simulink model "BMS_V4"  (R2017b)
settings: Solver=FixedStepDiscrete  StartTime=0.0  StopTime=inf  FixedStep=BASETIME  RelTol=1e-3  EnableMultiTasking=on
values from neighbouring files (symbols this model uses):
  AKT_BALANCE = uint16(8)    [BMS_V4_config.m]
  BALANCE = uint16(4)    [BMS_V4_config.m]
  BALANCE_RESISTOR = int32(5)    [BMS_V4_config.m]
  BALANCE_VEC = uint16(8)    [BMS_V4_config.m]
  CELL_SOC = uint16(7)    [BMS_V4_config.m]
  CELL_STATE = uint16(3)    [BMS_V4_config.m]
  CELL_TEMPERATURE = uint16(6)    [BMS_V4_config.m]
  CELL_VOLTAGE = uint16(5)    [BMS_V4_config.m]
  CELLACTBITFIELD = hex2dec('300')    [BMS_V4_config.m]
  CELLDEACTBITFIELD = hex2dec('100')    [BMS_V4_config.m]
  CELLT_BURST = uint16(6)    [BMS_V4_config.m]
  CELLV_BURST = uint16(5)    [BMS_V4_config.m]
  CLK_CYC_timer_1 = 586    [BMS_V4_config.m]
  CLK_CYC_timer_2 = 5860    [BMS_V4_config.m]
  CLK_CYC_timer_3 = 280    [BMS_V4_config.m]
  CLK_CYC_timer_4 = 586*100    (= 58600)    [BMS_V4_config.m]
  CLK_CYC_timer_5 = 5800*2    (= 11600)    [BMS_V4_config.m]
  CLK_CYC_timer_6 = 320    [BMS_V4_config.m]
  CN_CELLS = int32(40*3600)    [BMS_V4_config.m]
  CONTACTOR = uint16(1)    [BMS_V4_config.m]
  CONTACTOR_LOCKED = uint16(0)    [BMS_V4_config.m]
  CONTACTOR_UNLOCKED = uint16(1)    [BMS_V4_config.m]
  DEBUG_SEND_STATES = uint16(hex2dec('01'))    [BMS_V4_config.m]
  DELTA_SOC_BALANCE = int32(5*1e6)    [BMS_V4_config.m]
  DELTA_SOC_BALANCE_OFF = int32(1*1e5)    [BMS_V4_config.m]
  DETERMINE_MODEL_PARAMETER_ACT = uint16(100)    [BMS_V4_config.m]
  DETERMINE_MODEL_PARAMETER_SCC = uint16(101)    [BMS_V4_config.m]
  ERROR = uint16(1)    [BMS_V4_config.m]
  EXTERN_SIGNALS = uint16(1)    [BMS_V4_config.m]
  FREQUENCY_STEPS = uint16([25 50 75 100 150 250 500 750                                      1000 1500 2500 5000 7500                                      10010 10015 10025 10050 10075                                      10100 10150 10250 10500 10750                                      11000 11500])    [BMS_V4_config.m]
  GET_IMAG_PART_MFC = uint16(9)    [BMS_V4_config.m]
  GET_IMAG_PART_MSF = uint16(4)    [BMS_V4_config.m]
  GET_REAL_PART_MFC = uint16(8)    [BMS_V4_config.m]
  GET_REAL_PART_MSF = uint16(3)    [BMS_V4_config.m]
  IMU = uint16(7)    [BMS_V4_config.m]
  IMU_AMP_OFF = uint16(5)    [BMS_V4_config.m]
  IMU_DATA_READ_LOCUS_ACT = uint16(6)    [BMS_V4_config.m]
  IMU_DATA_READ_LOCUS_SCC = uint16(7)    [BMS_V4_config.m]
  IMU_DEBUG = uint16(9)    [BMS_V4_config.m]
  IMU_GET_DATA_MFC = uint16(8)    [BMS_V4_config.m]
  IMU_GET_DATA_MSF = uint16(3)    [BMS_V4_config.m]
  IMU_OFFSET_POLLING = uint16(11)    [BMS_V4_config.m]
  IMU_POLLING = uint16(2)    [BMS_V4_config.m]
  IMU_POWER = uint16(10)    [BMS_V4_config.m]
  IMU_SEND_IMAG = uint16(11)    [BMS_V4_config.m]
  IMU_SEND_REAL = uint16(10)    [BMS_V4_config.m]
  INDEX_IMAGPART = uint16(2)    [BMS_V4_config.m]
  INDEX_REALPART = uint16(1)    [BMS_V4_config.m]
  INFO = uint16(2)    [BMS_V4_config.m]
  INIT_OFFSET_AMPLITUDE = uint16(2)    [BMS_V4_config.m]
  LINE_CURRENT = uint16(3)    [BMS_V4_config.m]
  LINE_CURRENT_CANA = uint16(4)    [BMS_V4_config.m]
  LINE_CURRENT_SWITCH_THRESHOLD = int32(2*1e6)    [BMS_V4_config.m]
  NUM_OF_CELLS = uint16(16)    [BMS_V4_config.m]
  NUM_OF_FREQUENCIES_PSO = uint16(14)    [BMS_V4_config.m]
  NUM_OF_LINES = uint16(1)    [BMS_V4_config.m]
  NUM_OF_PARAMETER = single(5)    [BMS_V4_config.m]
  NUM_OF_SOC_POINTS = uint16(110)    [BMS_V4_config.m]
  P_L_BOUND = single([0.05;0.01;0.1;0.01;0.1])    [BMS_V4_config.m]
  P_U_BOUND = single([0.50;0.20;0.9;0.06;60])    [BMS_V4_config.m]
  PARA_ACT_SEND = uint16(101)    [BMS_V4_config.m]
  PARA_DATA_STORE_ACT = uint16(8)    [BMS_V4_config.m]
  PARA_DATA_STORE_SCC = uint16(9)    [BMS_V4_config.m]
  PARA_SCC_SEND = uint16(102)    [BMS_V4_config.m]
  PARTICLE_INIT = single(create_startparticle(P_L_BOUND,P_U_BOUND,NUM_OF_PARTICLE))    [BMS_V4_config.m]
  POLACT = hex2dec('00000BFF')    [BMS_V4_config.m]
  POLDEACT = hex2dec('000008FF')    [BMS_V4_config.m]
  PSO_PARA_DEBUG = uint16(13)    [BMS_V4_config.m]
  REQUEST_SOC_REF = uint16(1000)    [BMS_V4_config.m]
  SCALE_FACTOR_CH1 = single(0.66666666)    [BMS_V4_config.m]
  SCALE_FACTOR_CH2 = single(0.66666666)    [BMS_V4_config.m]
  SEND_CELL_SOC_ABS = uint16(199)    [BMS_V4_config.m]
  SHUT_DOWN_BALANCE_OFF = uint16(3)    [BMS_V4_config.m]
  SHUT_DOWN_BALANCE_ON = uint16(2)    [BMS_V4_config.m]
  START_IMU_MSL = uint16(3)    [BMS_V4_config.m]
  START_IMU_SCC = uint16(1)    [BMS_V4_config.m]
  SWITCH_IMU_OFF = uint16(2)    [BMS_V4_config.m]
  SWITCH_IMU_ON = uint16(1)    [BMS_V4_config.m]
  SWITCH_IMU_ON_OFF = uint16(4)    [BMS_V4_config.m]
  SYSTEM_DEBUG = uint16(12)    [BMS_V4_config.m]
  TIMEOUT_CANA = uint32(5000)    [BMS_V4_config.m]
  TIMEOUT_GATEWAY = uint32(500)    [BMS_V4_config.m]
  TS_SOC = single(0.010)    [BMS_V4_config.m]
  WARNING = uint16(2)    [BMS_V4_config.m]
libraries: c280xlib x44, c2833xlib x5, simulink x2, c2000lib x1, idelinklib_common x1
(part 6 of 8)

== stateflow chart BMS_V4/IMU_control ==
  state IMU
    state IMU_control [parallel]
      settings: executionOrder=1
      state init_
        en:
        imu_state=uint16(IMU_INIT);
        //imu_function = uint16(0);
      state IMU_start_slave
        state power_on_imu
          en:
          imu_state = IMU_POWER_ON;
          //balance disable
          imu_request = IMU_POWER;
          imu_in_progress=true;
          [imu_CAN_low, imu_CAN_high] = IMU_on_off(SWITCH_IMU_ON);
          gateway_request[IMU - uint16(1)] = true;
        state wait
          en:
        state init_offset_amplitude
          en:
          imu_on_off = true;
          imu_state = IMU_INIT_AMP_OFF;
          imu_request = IMU_AMP_OFF;
          [imu_CAN_low, imu_CAN_high] = IMU_set_offset_amplitude(imu_offset,imu_amplitude);
          //[imu_CAN_low, imu_CAN_high] = IMU_set_offset_amplitude(uint16(2000),uint16(500));
          gateway_request[IMU - uint16(1)] = true;
        power_on_imu -> wait : [imu_request_succed == true]
            | //clear MSG flag
            | {imu_request_succed = false;
            | imu_on_off = true;}
        wait -> init_offset_amplitude : after(TIMER_IMU_START_UP,sec)
      state reset
        imu_function = uint16(0);
      state IMU_msl
        // meas single locus
        state set_offset_on
          en:
          imu_state=MSL_SWITCH_OFFSET_ON;
          offset_flag = SWITCH_OFFSET_ON;
          send(IMU_OFFSET,IMU.IMU_offset_on_off);
        state time_for_transient_response
          en:
        state start_locus_measurement
          en:
          IMU_save_act_imu_soc();
          imu_state = MSL_START_LOCUS_MEAS;
          send(IMU_MEAS_LOCUS,IMU.IMU_meas_locus);
        state set_offset_off
          en:
          imu_state=MSL_SWITCH_OFFSET_OFF;
          offset_flag = SWITCH_OFFSET_OFF;
          send(IMU_OFFSET,IMU.IMU_offset_on_off);
        IMU.IMU_control.IMU_msl.set_offset_on -> IMU.IMU_control.IMU_msl.time_for_transient_response : [imu_offset_adjust  == true]
            | //clear MSG flag
            | {imu_offset_adjust = false;
            | imu_offset_is_set = true;}
        IMU.IMU_control.IMU_msl.time_for_transient_response -> start_locus_measurement : //after(TIMER_OFFSET_TRANSIENT_RESPONSE,sec)
            | after(40,sec)
        start_locus_measurement -> IMU.IMU_control.IMU_msl.set_offset_off : [imu_locus_ready == true]
            | {imu_locus_ready=false;}
      state IMU_nsr
        // start new state-of-charge reference
      state IMU_scc
        // start self calibrating cycle
        state set_offset_on
          en:
          imu_state=SCC_SWITCH_OFFSET_ON;
          offset_flag = SWITCH_OFFSET_ON;
          send(IMU_OFFSET,IMU.IMU_offset_on_off);
        state time_for_transient_response
          en:
          imu_cc_scc = int32(100*1e6);
          soc_point_counter = uint16(0);
        state meas_locus_at_actual_soc_point
          en:
          //scc_actual_soc_point = int32(imu_cc_scc);
          //scc_actual_soc_point = soc_point_counter;
          soc_points_of_scc[soc_point_counter] =  int32(imu_cc_scc);
          last_soc_point_index =  soc_point_counter + uint16(1); //simulink 1-indexing
          imu_state = SCC_START_LOCUS_MEAS;
          send(IMU_MEAS_LOCUS,IMU.IMU_meas_locus);
        state check_delta_SOC
          en:
          delta_SoC = int32(0);
          imu_state = SCC_CHECK_DELTA_SOC;
          du:
          delta_SoC = int32(soc_points_of_scc[soc_point_counter] - imu_cc_scc);
        state meas_last_locus [commented out]
          en:
          scc_actual_soc_point = imu_cc_scc;
          imu_state = SCC_MEAS_LAST_LOCUS;
          send(IMU_MEAS_LOCUS,IMU.IMU_meas_locus);
        state set_offset_off
          en:
          imu_state=SCC_SWITCH_OFFSET_OFF;
          offset_flag = SWITCH_OFFSET_OFF;
          send(IMU_OFFSET,IMU.IMU_offset_on_off);
        state store_soc_point_index
          en:
          mram_command[STORE_LAST_SOC_INDEX_SCC-uint16(1)]=true;
        state store_socpoints_scc
          en:
          mram_command[SOC_SCC_STORE-uint16(1)]=true;
        IMU.IMU_control.IMU_scc.set_offset_on -> IMU.IMU_control.IMU_scc.time_for_transient_response : [imu_offset_adjust  == true]
            | //clear MSG flag
            | {imu_offset_adjust = false;
            | imu_offset_is_set = true;}
        IMU.IMU_control.IMU_scc.time_for_transient_response -> meas_locus_at_actual_soc_point : after(TIMER_OFFSET_TRANSIENT_RESPONSE,sec)
        check_delta_SOC -> meas_locus_at_actual_soc_point [order 2] : [delta_SoC > SOC_STEP_SCC]
            | {soc_point_counter++;}
        meas_locus_at_actual_soc_point -> check_delta_SOC : [imu_locus_ready == true]
            | {imu_locus_ready=false;}
        check_delta_SOC -> IMU.IMU_control.IMU_scc.set_offset_off [order 1] : [min_cell_voltage < SCC_MIN_CELL_VOLTAGE]
        meas_last_locus -> IMU.IMU_control.IMU_scc.set_offset_off [commented out] : [imu_locus_ready == true]
            | {imu_locus_ready=false;}
        IMU.IMU_control.IMU_scc.set_offset_off -> store_soc_point_index : [imu_offset_adjust == true]
            | //clear MSG flag
            | {imu_offset_adjust = false;
            | imu_offset_is_set =false;}
        store_soc_point_index -> store_socpoints_scc : [mram_command[STORE_LAST_SOC_INDEX_SCC-uint16(1)] == false]
      state IMU_stop_slave
        state safty_wait
        state power_off_imu
          en:
          imu_state = IMU_POWER_OFF;
          //balance enable
          imu_request = IMU_POWER;
          [imu_CAN_low, imu_CAN_high] = IMU_on_off(SWITCH_IMU_OFF);
          gateway_request[IMU - uint16(1)] = true;
        safty_wait -> power_off_imu : after(TIMER_IMU_START_UP,sec)
      (junction 13) -> IMU.IMU_control.IMU_scc.set_offset_on [order 1] : [imu_function == START_IMU_SCC]
          | {imu_scc_finish = false;}
          | // start self calibration cycle
      store_socpoints_scc -> (junction 106) : [mram_command[SOC_SCC_STORE-uint16(1)] == false]
          | {imu_scc_finish = true;}
      IMU.IMU_control.IMU_msl.set_offset_off -> (junction 106) : [imu_offset_adjust == true]
          | //clear MSG flag
          | {imu_offset_adjust = false;
          | imu_offset_is_set =false;}
      (default) -> init_
      init_ -> power_on_imu : [ imu_function!=0 ]
          | {imu_finish=false;}
      reset -> init_
      (junction 13) -> IMU.IMU_control.IMU_msl.set_offset_on [order 3] : [imu_function == START_IMU_MSL]
          | // meas single locus
      (junction 13) -> IMU_nsr [order 2] : [imu_function == START_IMU_NSR]
          | // start new state-of-charge reference
      (junction 37) -> reset : {imu_function = uint16(0);
          | imu_in_progress=false;
          | imu_finish=true;}
      power_off_imu -> (junction 37) : [imu_request_succed == true]
          | //clear MSG flag
          | {imu_request_succed = false;
          | imu_on_off = false;}
      IMU_nsr -> (junction 106)
      (junction 106) -> safty_wait
      init_offset_amplitude -> (junction 13) : [imu_request_succed == true]
          | //clear MSG flag
          | {imu_request_succed = false;}
    state IMU_meas_locus [parallel]
      // control for measurement and storage of one locus
      settings: executionOrder=2
      state init
      state frequency_single_measurement
      state frequency_collective_measurement
        state start_mfc
          en:
          imu_state=IMU_MFC_START;
          freq_index=uint16(0);
          act_cellNo=uint16(0);
          act_lineNo=uint16(0);
          send(IMU_MFC,IMU.IMU_mfc);
        state get_data_mfc
          en:
          imu_state = IMU_MFC_GET_DATA;
          imu_request = IMU_GET_DATA_MFC;
          [imu_CAN_low, imu_CAN_high]=IMU_get_data_mfc(act_lineNo,act_cellNo,freq_index);
          gateway_request[ IMU - uint16(1)] = true;
        state store_data
          en:
          imu_state = IMU_MFC_STORE_DATA;
          send(IMU_STORE_DATA,IMU.IMU_store_data);
        start_mfc -> get_data_mfc : IMU_MFC_READY
        (junction 262) -> get_data_mfc
        get_data_mfc -> store_data : [imu_request_succed == true]
            | //clear MSG flag
            | {imu_request_succed = false;}
        (junction 265) -> (junction 262)
        (junction 261) -> (junction 265)
        (junction 241) -> (junction 262) [order 1] : //[act_cellNo < NUM_OF_CELLS]
            | [freq_index < NUM_OF_FREQUENCIES]
        store_data -> (junction 239) : [imu_store_ready==true]
            | {imu_store_ready=false;
            | freq_index++;}
            | //act_cellNo++;}
        (junction 241) -> (junction 261) [order 2] : //[ (act_cellNo >= NUM_OF_CELLS) &&  ( freq_index < (NUM_OF_FREQUENCIES-uint16(1))) ]
            | //Attention NUM_OF_FREQUENCIES -1 after this freq_index is incremented!!
            | [ (freq_index >= NUM_OF_FREQUENCIES) &&  ( act_cellNo < (NUM_OF_CELLS-uint16(1))) ]
            | {act_cellNo++;
            | freq_index=uint16(0);}
            | //freq_index++;
            | //act_cellNo=uint16(0);
            | //act_lineNo=uint16(0);}
        (junction 239) -> (junction 241)
      (default) -> IMU.IMU_meas_locus.init
      (junction 117) -> frequency_single_measurement [order 2] : [imu_meas_method==MSF]
          | // not yet implemented
      IMU.IMU_meas_locus.init -> (junction 117) : IMU_MEAS_LOCUS
      (junction 117) -> start_mfc [order 1] : [imu_meas_method==MFC]
          | // implemented
      (junction 270) -> IMU.IMU_meas_locus.init
      frequency_single_measurement -> (junction 273)
      (junction 268) -> (junction 270)
      (junction 273) -> (junction 268)
      (junction 241) -> (junction 268) [order 3] : //[ freq_index >= (NUM_OF_FREQUENCIES-uint16(1))]
          | [ act_cellNo >= (NUM_OF_CELLS -uint16(1)) ]
          | {imu_locus_ready = true;}
    state IMU_mfc [parallel]
      // meas frequency collective
      settings: executionOrder=3
      state send_start_mfc
        en:
        imu_mfc_state = MFC_START;
        imu_request = IMU_START_MFC;
        [imu_CAN_low , imu_CAN_high]= IMU_start_mfc(FREQUENCY_STEPS[uint16(0)],FREQUENCY_ID);
        gateway_request[ IMU - uint16(1)] = true;
      state init
        en:
        imu_mfc_state=MFC_INIT;
        imu_mfc_ready =false;
      state waiting
      state wait_for_polling
        en:
        imu_mfc_state = MFC_POLLING;
      state polling
        en:
        imu_mfc_state = MFC_POLLING;
        imu_request  = IMU_POLLING;
        imu_CAN_low = uint32(IMU_POLLING);
        imu_CAN_high = uint32(0);
        gateway_request[ IMU - uint16(1)] = true;
      (default) -> IMU.IMU_mfc.init
      IMU.IMU_mfc.init -> IMU.IMU_mfc.waiting : IMU_MFC
      IMU.IMU_mfc.waiting -> send_start_mfc : after(1,sec)
      (junction 173) -> IMU.IMU_mfc.init [order 2] : //MAESUREMENT_FINISH
          | [imu_mfc_ready == true]
          | {send(IMU_MFC_READY,IMU.IMU_meas_locus);}
      send_start_mfc -> IMU.IMU_mfc.wait_for_polling : [imu_request_succed == true]
          | //clear MSG flag
          | {imu_request_succed = false;}
      (junction 173) -> IMU.IMU_mfc.wait_for_polling [order 1] : [imu_mfc_ready == false]
      IMU.IMU_mfc.wait_for_polling -> IMU.IMU_mfc.polling : after(TIMER_IMU_POLLING,sec)
      IMU.IMU_mfc.polling -> (junction 173) : [imu_request_succed == true]
          | //clear MSG flag
          | {imu_request_succed = false;}
    state IMU_store_data [parallel]
      settings: executionOrder=4
      state init
      state store_to_MRAM_scc
        //imu_state
        cell_No = uint16(imu_act_cellno);
        line_No = uint16(imu_act_lineno);
        freq_ind = uint16(imu_act_freq_index);
        imu_act_soc = soc_points_of_scc[soc_point_counter]
      state store_to_MRAM_act
        //imu_state
        cell_No = uint16(imu_act_cellno);
        line_No = uint16(imu_act_lineno);
        freq_ind = uint16(imu_act_freq_index);
        imu_act_soc = soc_of_locus_set[cell_No-uint16(1) ];
      state store_to_mram
        en:
        mram_command[IMU_DATA_STORE- uint16(1)] = true;
      state send_can_cell_imu_real_part
        en:
        [imu_debug_CAN_low,imu_debug_CAN_high]=IMU_debug_send_cell_real(cell_No,freq_ind,imu_act_soc,imu_act_realpart);
        CANA_send_data[IMU_SEND_REAL - uint16(1)] = true;
      state send_can_cell_imu_imag_part
        en:
        [imu_debug_CAN_low,imu_debug_CAN_high]=IMU_debug_send_cell_imag(cell_No,freq_ind,imu_act_soc,imu_act_imagpart);
        CANA_send_data[IMU_SEND_IMAG - uint16(1)] = true;
      IMU.IMU_store_data.init -> (junction 410) : IMU_STORE_DATA
      (default) -> IMU.IMU_store_data.init
      (junction 410) -> store_to_MRAM_scc [order 1] : [imu_function == START_IMU_SCC]
      (junction 410) -> store_to_MRAM_act [order 2] : [imu_function == START_IMU_MSL]
      send_can_cell_imu_imag_part -> IMU.IMU_store_data.init : after(TIMER_IMU_DEBUG_SEND_DATA,sec)
          | [CANA_send_data[IMU_SEND_IMAG - uint16(1)] == false]
          | {imu_store_ready = true;
          | imu_send_meas_data = false;}
      store_to_MRAM_scc -> store_to_mram
      store_to_MRAM_act -> store_to_mram
      store_to_mram -> send_can_cell_imu_real_part : [mram_command[IMU_DATA_STORE- uint16(1)] == false]
          | {imu_send_meas_data = true;}
      send_can_cell_imu_real_part -> send_can_cell_imu_imag_part : after(TIMER_IMU_DEBUG_SEND_DATA,sec)
          | [CANA_send_data[IMU_SEND_REAL - uint16(1)] == false]
    state IMU_offset_on_off [parallel]
      // meas frequency collective
      settings: executionOrder=5
      state switch_offset_on_or_off
        en:
        //imu_mfc_state = MFC_START;
        imu_request = IMU_OFFSET_ON_OFF;
        [imu_CAN_low , imu_CAN_high] = IMU_switch_offset_on_off(offset_flag);
        gateway_request[ IMU - uint16(1)] = true;
      state init
        en:
        //imu_mfc_state=MFC_INIT;
        //imu_offset_ready = false;
      state waiting
      state wait_for_polling
        en:
        //imu_mfc_state = MFC_POLLING;
      state polling
        en:
        //imu_mfc_state = MFC_POLLING;
        imu_request  = IMU_OFFSET_POLLING; // different polling code "11" for handle imu_RX
        imu_CAN_low = uint32(IMU_POLLING); // polling always code "2"
        imu_CAN_high = uint32(0);
        gateway_request[ IMU - uint16(1)] = true;
      (default) -> IMU.IMU_offset_on_off.init
      IMU.IMU_offset_on_off.init -> IMU.IMU_offset_on_off.waiting : IMU_OFFSET
      IMU.IMU_offset_on_off.waiting -> switch_offset_on_or_off : after(1,sec)
      (junction 332) -> IMU.IMU_offset_on_off.init [order 2] : //MAESUREMENT_FINISH
          | [imu_offset_ready == true]
          | {imu_offset_adjust = true;...
          | imu_offset_ready = false;}
          | //{imu_request_succed = true;}
          | //{send(IMU_OFFSET_READY,IMU.IMU_control);}
      switch_offset_on_or_off -> IMU.IMU_offset_on_off.wait_for_polling : [imu_request_succed == true]
          | //clear MSG flag
          | {imu_request_succed = false;}
      (junction 332) -> IMU.IMU_offset_on_off.wait_for_polling [order 1] : [imu_offset_ready == false]
      IMU.IMU_offset_on_off.wait_for_polling -> IMU.IMU_offset_on_off.polling : after(TIMER_IMU_POLLING,sec)
      IMU.IMU_offset_on_off.polling -> (junction 332) : [imu_request_succed == true]
          | //clear MSG flag
          | {imu_request_succed = false;}
  data: CAN_LOW function_output uint32; CAN_HIGH function_output uint32; on_off function_input uint16; CAN_LOW function_output uint32; CAN_HIGH function_output uint32; offset function_input uint16; amplitude function_input uint16; CAN_LOW function_output uint32; CAN_HIGH function_output uint32; offset_on_off function_input uint16; start_frequency function_input uint16; frequency_ID function_input uint16; CAN_LOW function_output uint32; CAN_HIGH function_output uint32; lineNo function_input uint16; cellNo function_input uint16; frequency_index function_input uint16; CAN_LOW function_output uint32; CAN_HIGH function_output uint32; cellNo function_input uint16; freq_id function_input uint16; soc function_input int32; cell_real_part function_input single; CAN_LOW function_output uint32; CAN_HIGH function_output uint32; cellNo function_input uint16; freq_id function_input uint16; soc function_input int32; cell_imag_part function_input single; CAN_LOW function_output uint32; CAN_HIGH function_output uint32; imu_state data_store_memory; IMU_INIT parameter; START_IMU_SCC parameter; START_IMU_NSR parameter uint16; START_IMU_MSL parameter; imu_function data_store_memory; imu_request_succed data_store_memory; imu_offset_is_set data_store_memory; imu_request data_store_memory; IMU_POWER parameter; imu_CAN_high data_store_memory; imu_CAN_low data_store_memory; TIMER_IMU_START_UP parameter; imu_on_off data_store_memory; IMU_POWER_ON parameter; SWITCH_IMU_ON parameter; SWITCH_IMU_OFF parameter; IMU parameter; gateway_request data_store_memory; IMU_INIT_AMP_OFF parameter; IMU_AMP_OFF parameter; imu_offset data_store_memory; imu_amplitude data_store_memory; SWITCH_OFFSET_ON parameter; SWITCH_OFFSET_OFF parameter; MSL_SWITCH_OFFSET_ON parameter; imu_locus_ready local boolean =false; IMU_MFC_START parameter; imu_act_soc data_store_memory; cell_soc_CC data_store_memory; MFC_START parameter; MFC_INIT parameter; imu_mfc_state data_store_memory; IMU_START_MFC parameter; FREQUENCY_ID parameter; FREQUENCY_STEPS parameter; NUM_OF_FREQUENCIES parameter; MFC_POLLING parameter; TIMER_IMU_POLLING parameter; IMU_POLLING parameter; imu_mfc_ready data_store_memory; imu_act_freq_index data_store_memory; act_cellNo local uint16; act_lineNo local uint16; freq_index local uint16; IMU_MFC_GET_DATA parameter; MSL_START_LOCUS_MEAS parameter; MSL_SWITCH_OFFSET_OFF parameter; MSF parameter; MFC parameter; imu_meas_method data_store_memory; IMU_MFC_STORE_DATA parameter; imu_debug_CAN_low data_store_memory; imu_debug_CAN_high data_store_memory; DEBUG_CELL_INFO parameter; DEBUG_CELL_REAL parameter; DEBUG_CELL_IMAG parameter; imu_act_cellno data_store_memory; imu_act_lineno data_store_memory; IMU_GET_DATA_MFC parameter; TIMER_IMU_DEBUG_SEND_DATA parameter; CANA_send_data data_store_memory; IMU_DEBUG parameter; imu_store_ready local boolean =false; NUM_OF_CELLS parameter; NUM_OF_LINES parameter; imu_act_imagpart data_store_memory; imu_act_realpart data_store_memory; IMU_POWER_OFF parameter; imu_send_meas_data data_store_memory; imu_in_progress data_store_memory; IMU_OFFSET_ON_OFF parameter; imu_finish data_store_memory; cell_No local uint16; freq_ind local uint16; line_No local uint16; act_soc local int32; IMU_SEND_REAL parameter; IMU_SEND_IMAG parameter; IMU_DATA_STORE parameter; mram_command data_store_memory; soc_of_locus_set data_store_memory; IMU_OFFSET_POLLING parameter; imu_offset_ready data_store_memory; offset_flag local uint16; imu_offset_adjust local boolean; imu_cc_scc data_store_memory; min_cell_voltage data_store_memory; delta_SoC local int32; imu_scc_finish data_store_memory; SCC_CHECK_DELTA_SOC parameter; SCC_MEAS_LAST_LOCUS parameter; SCC_MIN_CELL_VOLTAGE parameter; SCC_START_LOCUS_MEAS parameter; SCC_SWITCH_OFFSET_OFF parameter; SCC_SWITCH_OFFSET_ON parameter; SOC_STEP_SCC parameter; TIMER_OFFSET_TRANSIENT_RESPONSE parameter; SOC_SCC_STORE parameter; soc_points_of_scc data_store_memory; soc_point_counter data_store_memory; last_soc_point_index data_store_memory; STORE_LAST_SOC_INDEX_SCC parameter
  events: trigger_IMU input FUNCTION_CALL_EVENT; IMU_MEAS_LOCUS local FUNCTION_CALL_EVENT; IMU_MFC local FUNCTION_CALL_EVENT; IMU_MFC_READY local FUNCTION_CALL_EVENT; IMU_STORE_DATA local FUNCTION_CALL_EVENT; IMU_OFFSET local FUNCTION_CALL_EVENT; IMU_OFFSET_READY local FUNCTION_CALL_EVENT
  function [CAN_LOW,CAN_HIGH]=IMU_on_off(on_off):
    | function [CAN_LOW,CAN_HIGH]=IMU_on_off(on_off)
    | 
    | CODE = uint16([IMU_POWER 0 0 0]);
    | 
    | switch on_off
    |     case SWITCH_IMU_ON
    |        CODE(2) = SWITCH_IMU_ON; %IMU ON  
    |     case SWITCH_IMU_OFF
    |        CODE(2) = SWITCH_IMU_OFF; %IMU OFF    
    | end
    | 
    | x1=uint16(bitand(uint16(hex2dec('00ff')),uint16(CODE(1))));
    | x2=uint16(bitand(uint16(hex2dec('ff00')),uint16(bitshift(uint16(CODE(2)),8))));
    | x3=uint16(bitand(uint16(hex2dec('00ff')),uint16(CODE(3))));
    | x4=uint16(bitand(uint16(hex2dec('ff00')),uint16(bitshift(uint16(CODE(4)),8))));
    | 
    | x11=uint16(bitor(x1,x2));
    | x12=uint16(bitor(x3,x4));
    | 
    | out1=uint32(bitor(uint32(x11),bitshift(uint32(x12),16)));
    | 
    | CAN_LOW=out1;
    | CAN_HIGH=uint32(0);
    | end
  function [CAN_LOW,CAN_HIGH]=IMU_set_offset_amplitude(offset, amplitude):
    | function [CAN_LOW,CAN_HIGH]=IMU_set_offset_amplitude(offset, amplitude)
    | 
    | CODE = uint16([IMU_AMP_OFF 0 0 0 0 0 0 0]);
    | 
    | CODE(2)= uint16(bitand(uint16(hex2dec('00ff')),uint16(offset)));
    | CODE(3)= uint16(bitand(uint16(hex2dec('00ff')),bitshift(uint16(offset),-8)));
    | CODE(4)= uint16(bitand(uint16(hex2dec('00ff')),uint16(amplitude)));
    | CODE(5)= uint16(bitand(uint16(hex2dec('00ff')),bitshift(uint16(amplitude),-8)));
    | 
    | x1=uint16(bitand(uint16(hex2dec('00ff')),uint16(CODE(1))));
    | x2=uint16(bitand(uint16(hex2dec('ff00')),uint16(bitshift(uint16(CODE(2)),8))));
    | x3=uint16(bitand(uint16(hex2dec('00ff')),uint16(CODE(3))));
    | x4=uint16(bitand(uint16(hex2dec('ff00')),uint16(bitshift(uint16(CODE(4)),8))));
    | 
    | x11=uint16(bitor(x1,x2));
    | x12=uint16(bitor(x3,x4));
    | 
    | out1=uint32(bitor(uint32(x11),bitshift(uint32(x12),16)));
    | 
    | 
    | x5=uint16(bitand(uint16(hex2dec('00ff')),uint16(CODE(5))));
    | x6=uint16(bitand(uint16(hex2dec('ff00')),uint16(bitshift(uint16(CODE(6)),8))));
    | x7=uint16(bitand(uint16(hex2dec('00ff')),uint16(CODE(7))));
    | x8=uint16(bitand(uint16(hex2dec('ff00')),uint16(bitshift(uint16(CODE(8)),8))));
    | 
    | x21=uint16(bitor(x5,x6));
    | x22=uint16(bitor(x7,x8));
    | 
    | out2=uint32(bitor(uint32(x21),bitshift(uint32(x22),16)));
    | 
    | CAN_LOW=out1;
    | CAN_HIGH=out2;
    | end
  function [CAN_LOW,CAN_HIGH]=IMU_switch_offset_on_off(offset_on_off):
    | function [CAN_LOW,CAN_HIGH]=IMU_switch_offset_on_off(offset_on_off)
    | 
    | CODE = uint16([IMU_OFFSET_ON_OFF 0 0 0]);
    | 
    | switch offset_on_off
    |     case SWITCH_OFFSET_ON
    |        CODE(2) = SWITCH_OFFSET_ON; %OFFSET ON  
    |     case SWITCH_OFFSET_OFF
    |        CODE(2) = SWITCH_OFFSET_OFF; %OFFSET OFF    
    | end
    | 
    | x1=uint16(bitand(uint16(hex2dec('00ff')),uint16(CODE(1))));
    | x2=uint16(bitand(uint16(hex2dec('ff00')),uint16(bitshift(uint16(CODE(2)),8))));
    | x3=uint16(bitand(uint16(hex2dec('00ff')),uint16(CODE(3))));
    | x4=uint16(bitand(uint16(hex2dec('ff00')),uint16(bitshift(uint16(CODE(4)),8))));
    | 
    | x11=uint16(bitor(x1,x2));
    | x12=uint16(bitor(x3,x4));
    | 
    | out1=uint32(bitor(uint32(x11),bitshift(uint32(x12),16)));
    | 
    | CAN_LOW=out1;
    | CAN_HIGH=uint32(0);
    | end
  function [CAN_LOW,CAN_HIGH]=IMU_start_mfc(start_frequency, frequency_ID):
    | function [CAN_LOW,CAN_HIGH]=IMU_start_mfc(start_frequency, frequency_ID)
    | 
    | CODE = uint16([IMU_START_MFC 0 0 0 0 0 0 0]);
    | 
    | CODE(2)= uint16(bitand(uint16(hex2dec('00ff')),uint16(start_frequency)));
    | CODE(3)= uint16(bitand(uint16(hex2dec('00ff')),bitshift(uint16(start_frequency),-8)));
    | CODE(4)= uint16(bitand(uint16(hex2dec('00ff')),uint16(frequency_ID)));
    | 
    | x1=uint16(bitand(uint16(hex2dec('00ff')),uint16(CODE(1))));
    | x2=uint16(bitand(uint16(hex2dec('ff00')),uint16(bitshift(uint16(CODE(2)),8))));
    | x3=uint16(bitand(uint16(hex2dec('00ff')),uint16(CODE(3))));
    | x4=uint16(bitand(uint16(hex2dec('ff00')),uint16(bitshift(uint16(CODE(4)),8))));
    | 
    | x11=uint16(bitor(x1,x2));
    | x12=uint16(bitor(x3,x4));
    | 
    | out1=uint32(bitor(uint32(x11),bitshift(uint32(x12),16)));
    | 
    | 
    | x5=uint16(bitand(uint16(hex2dec('00ff')),uint16(CODE(5))));
    | x6=uint16(bitand(uint16(hex2dec('ff00')),uint16(bitshift(uint16(CODE(6)),8))));
    | x7=uint16(bitand(uint16(hex2dec('00ff')),uint16(CODE(7))));
    | x8=uint16(bitand(uint16(hex2dec('ff00')),uint16(bitshift(uint16(CODE(8)),8))));
    | 
    | x21=uint16(bitor(x5,x6));
    | x22=uint16(bitor(x7,x8));
    | 
    | out2=uint32(bitor(uint32(x21),bitshift(uint32(x22),16)));
    | 
    | 
    | CAN_LOW=out1;
    | CAN_HIGH=out2;
  function [CAN_LOW, CAN_HIGH]=IMU_get_data_mfc(lineNo,cellNo,frequency_index):
    | function [CAN_LOW, CAN_HIGH]=IMU_get_data_mfc(lineNo,cellNo,frequency_index)
    | 
    | CODE = uint16([IMU_GET_DATA_MFC 0 0 0 0 0 0 0]);
    | 
    | CODE(2)= uint16(bitand(uint16(hex2dec('00ff')),uint16(lineNo)));
    | CODE(3)= uint16(bitand(uint16(hex2dec('00ff')),uint16(cellNo)));
    | CODE(4)= uint16(bitand(uint16(hex2dec('00ff')),uint16(frequency_index)));
    | 
    | x1=uint16(bitand(uint16(hex2dec('00ff')),uint16(CODE(1))));
    | x2=uint16(bitand(uint16(hex2dec('ff00')),uint16(bitshift(uint16(CODE(2)),8))));
    | x3=uint16(bitand(uint16(hex2dec('00ff')),uint16(CODE(3))));
    | x4=uint16(bitand(uint16(hex2dec('ff00')),uint16(bitshift(uint16(CODE(4)),8))));
    | 
    | x11=uint16(bitor(x1,x2));
    | x12=uint16(bitor(x3,x4));
    | 
    | out1=uint32(bitor(uint32(x11),bitshift(uint32(x12),16)));
    | 
    | 
    | x5=uint16(bitand(uint16(hex2dec('00ff')),uint16(CODE(5))));
    | x6=uint16(bitand(uint16(hex2dec('ff00')),uint16(bitshift(uint16(CODE(6)),8))));
    | x7=uint16(bitand(uint16(hex2dec('00ff')),uint16(CODE(7))));
    | x8=uint16(bitand(uint16(hex2dec('ff00')),uint16(bitshift(uint16(CODE(8)),8))));
    | 
    | x21=uint16(bitor(x5,x6));
    | x22=uint16(bitor(x7,x8));
    | 
    | out2=uint32(bitor(uint32(x21),bitshift(uint32(x22),16)));
    | 
    | 
    | CAN_LOW=out1;
    | CAN_HIGH=out2;
  function IMU_save_act_imu_soc:
    | function IMU_save_act_imu_soc
    |  
    | global soc_of_locus_set;
    | global cell_soc_CC; 
    | 
    | soc_of_locus_set = cell_soc_CC(:,1);
  function [CAN_LOW, CAN_HIGH] = IMU_debug_send_cell_real(cellNo,freq_id,soc,cell_real_part):
    | function [CAN_LOW, CAN_HIGH] = IMU_debug_send_cell_real(cellNo,freq_id,soc,cell_real_part)
    |  
    | CODE = uint16([0 0 0 0 0 0 0 0]);
    | 
    | soc_s=single(soc);
    | soc_convert = typecast(soc/1e6,'uint32');  
    | soc1 = uint16(bitand(uint32(hex2dec('000000FF')),soc_convert));
    | frequence=FREQUENCY_STEPS(freq_id);
    | real_part=typecast(cell_real_part,'uint32');
    | 
    | CODE(1)= uint16(bitand(uint16(hex2dec('00ff')),uint16(cellNo)));
    | CODE(2)= uint16(bitand(uint16(hex2dec('00ff')),uint16(frequence)));
    | CODE(3)= uint16(bitand(uint16(hex2dec('00ff')),bitshift(uint16(frequence),-8)));
    | CODE(4)= uint16(bitand(uint16(hex2dec('00ff')),uint16(soc1)));
    | 
    | CODE(5)= uint16(bitand(uint32(hex2dec('000000ff')),real_part));
    | CODE(6)= uint16(bitand(uint32(hex2dec('000000ff')),bitshift(real_part,-8)));
    | CODE(7)= uint16(bitand(uint32(hex2dec('000000ff')),bitshift(real_part,-16)));
    | CODE(8)= uint16(bitand(uint32(hex2dec('000000ff')),bitshift(real_part,-24)));
    | 
    | x1=uint16(bitand(uint16(hex2dec('00ff')),uint16(CODE(1))));
    | x2=uint16(bitand(uint16(hex2dec('ff00')),uint16(bitshift(uint16(CODE(2)),8))));
    | x3=uint16(bitand(uint16(hex2dec('00ff')),uint16(CODE(3))));
    | x4=uint16(bitand(uint16(hex2dec('ff00')),uint16(bitshift(uint16(CODE(4)),8))));
    | 
    | x11=uint16(bitor(x1,x2));
    | x12=uint16(bitor(x3,x4));
    | 
    | out1=uint32(bitor(uint32(x11),bitshift(uint32(x12),16)));
    | 
    | x5=uint16(bitand(uint16(hex2dec('00ff')),uint16(CODE(5))));
    | x6=uint16(bitand(uint16(hex2dec('ff00')),uint16(bitshift(uint16(CODE(6)),8))));
    | x7=uint16(bitand(uint16(hex2dec('00ff')),uint16(CODE(7))));
    | x8=uint16(bitand(uint16(hex2dec('ff00')),uint16(bitshift(uint16(CODE(8)),8))));
    | 
    | x21=uint16(bitor(x5,x6));
    | x22=uint16(bitor(x7,x8));
    | 
    | out2=uint32(bitor(uint32(x21),bitshift(uint32(x22),16)));
    | 
    | CAN_LOW=out1;
    | CAN_HIGH=out2;
  function [CAN_LOW, CAN_HIGH] = IMU_debug_send_cell_imag(cellNo,freq_id,soc,cell_imag_part):
    | function [CAN_LOW, CAN_HIGH] = IMU_debug_send_cell_imag(cellNo,freq_id,soc,cell_imag_part)
    |  
    | CODE = uint16([0 0 0 0 0 0 0 0]);
    | 
    | soc_s=single(soc);
    | soc_convert = typecast(soc/1e6,'uint32');  
    | soc1 = uint16(bitand(uint32(hex2dec('000000FF')),soc_convert));
    | frequence=FREQUENCY_STEPS(freq_id);
    | imag_part=typecast(cell_imag_part,'uint32');
    | 
    | CODE(1)= uint16(bitand(uint16(hex2dec('00ff')),uint16(cellNo)));
    | CODE(2)= uint16(bitand(uint16(hex2dec('00ff')),uint16(frequence)));
    | CODE(3)= uint16(bitand(uint16(hex2dec('00ff')),bitshift(uint16(frequence),-8)));
    | CODE(4)= uint16(bitand(uint16(hex2dec('00ff')),uint16(soc1)));
    | 
    | CODE(5)= uint16(bitand(uint32(hex2dec('000000ff')),imag_part));
    | CODE(6)= uint16(bitand(uint32(hex2dec('000000ff')),bitshift(imag_part,-8)));
    | CODE(7)= uint16(bitand(uint32(hex2dec('000000ff')),bitshift(imag_part,-16)));
    | CODE(8)= uint16(bitand(uint32(hex2dec('000000ff')),bitshift(imag_part,-24)));
    | 
    | x1=uint16(bitand(uint16(hex2dec('00ff')),uint16(CODE(1))));
    | x2=uint16(bitand(uint16(hex2dec('ff00')),uint16(bitshift(uint16(CODE(2)),8))));
    | x3=uint16(bitand(uint16(hex2dec('00ff')),uint16(CODE(3))));
    | x4=uint16(bitand(uint16(hex2dec('ff00')),uint16(bitshift(uint16(CODE(4)),8))));
    | 
    | x11=uint16(bitor(x1,x2));
    | x12=uint16(bitor(x3,x4));
    | 
    | out1=uint32(bitor(uint32(x11),bitshift(uint32(x12),16)));
    | 
    | x5=uint16(bitand(uint16(hex2dec('00ff')),uint16(CODE(5))));
    | x6=uint16(bitand(uint16(hex2dec('ff00')),uint16(bitshift(uint16(CODE(6)),8))));
    | x7=uint16(bitand(uint16(hex2dec('00ff')),uint16(CODE(7))));
    | x8=uint16(bitand(uint16(hex2dec('ff00')),uint16(bitshift(uint16(CODE(8)),8))));
    | 
    | x21=uint16(bitor(x5,x6));
    | x22=uint16(bitor(x7,x8));
    | 
    | out2=uint32(bitor(uint32(x21),bitshift(uint32(x22),16)));
    | 
    | CAN_LOW=out1;
    | CAN_HIGH=out2;

== matlab function BMS_V4/FunctionCall_CANB_RX/handle_control_imu/control_imu_proceeding ==
  data: msg input; imu_request_succed data_store_memory; imu_request data_store_memory; IMU_GET_DATA_MSF parameter; GET_IMAG_PART_MSF parameter; GET_REAL_PART_MSF parameter; imu_act_cellno data_store_memory; imu_act_lineno data_store_memory; imu_act_imagpart data_store_memory; imu_act_realpart data_store_memory; next_gateway_request data_store_memory; IMU_POLLING parameter; imu_mfc_ready data_store_memory; IMU_GET_DATA_MFC parameter; GET_REAL_PART_MFC parameter; GET_IMAG_PART_MFC parameter; imu_act_freq_index data_store_memory; INDEX_REALPART parameter; INDEX_IMAGPART parameter; imu_amplitude data_store_memory; imu_offset data_store_memory; IMU_AMP_OFF parameter; IMU parameter; gateway_request data_store_memory; imu_offset_ready data_store_memory; IMU_OFFSET_POLLING parameter
function control_imu_proceeding(msg,IMU_GET_DATA_MSF,GET_IMAG_PART_MSF,...
    GET_REAL_PART_MSF,IMU_POLLING,IMU_GET_DATA_MFC,GET_REAL_PART_MFC,...
    GET_IMAG_PART_MFC,INDEX_REALPART,INDEX_IMAGPART,IMU_AMP_OFF,IMU,...
    IMU_OFFSET_POLLING)


global next_gateway_request;
global imu_request_succed;
global imu_request;
global imu_act_cellno;
global imu_act_lineno;
%global imu_act_soc;
global imu_act_imagpart;
global imu_act_realpart;
global imu_mfc_ready;
global imu_offset_ready;
global imu_act_freq_index;
% global one_locus_set;
global imu_amplitude;
global imu_offset;
global gateway_request;


imu_id = uint16(bitand(uint32(hex2dec('000000FF')),msg(1)));

if imu_request == IMU_GET_DATA_MSF %get data

    if imu_id == GET_REAL_PART_MSF %get real part
        imu_act_lineno = uint16(bitand(uint32(hex2dec('000000FF')),...
            bitshift(msg(1),-8)))+uint16(1);
        imu_act_cellno = uint16(bitand(uint32(hex2dec('000000FF')),...
            bitshift(msg(1),-16)))+uint16(1);
        cell_data = uint32(bitor(bitand(uint32(hex2dec('000000FF')),...
            bitshift(msg(1),-24)),bitand(uint32(hex2dec('FFFFFF00')),...
            bitshift(msg(2),8))));
        imu_act_realpart = typecast(cell_data,'single');
    end  
    if imu_id == GET_IMAG_PART_MSF %get imag part
        imu_act_lineno = uint16(bitand(uint32(hex2dec('000000FF')),...
            bitshift(msg(1),-8)))+uint16(1);
        imu_act_cellno = uint16(bitand(uint32(hex2dec('000000FF')),...
            bitshift(msg(1),-16)))+uint16(1);
        cell_data = uint32(bitor(bitand(uint32(hex2dec('000000FF')),...
            bitshift(msg(1),-24)),bitand(uint32(hex2dec('FFFFFF00')),...
            bitshift(msg(2),8))));
        imu_act_imagpart = typecast(cell_data,'single');
                
        imu_request_succed=true; % both received ready
%         gateway_request(IMU) = false;
        next_gateway_request =true;
    end
    
elseif imu_request == IMU_GET_DATA_MFC %get data
    
    act_line_no = uint16(bitand(uint32(hex2dec('000000FF')),...
           bitshift(msg(1),-8)))+uint16(1);
    act_cellno = uint16(bitand(uint32(hex2dec('000000FF')),...
           bitshift(msg(1),-16)))+uint16(1);
    act_freq_index = uint16(bitand(uint32(hex2dec('000000FF')),...
           bitshift(msg(1),-24)))+uint16(1);
    cell_data = uint32(msg(2));
    act_complexpart = typecast(cell_data,'single');
    
    if imu_id == GET_REAL_PART_MFC %get real part
        
        imu_act_lineno = act_line_no;
        imu_act_cellno = act_cellno;
        imu_act_freq_index = act_freq_index;
        imu_act_realpart = act_complexpart;       
%         one_locus_set(act_freq_index,INDEX_REALPART,act_cellno)=...
%             act_complexpart;
    end  
    if imu_id == GET_IMAG_PART_MFC %get imag part
        
        imu_act_lineno = act_line_no;
        imu_act_cellno = act_cellno;
        imu_act_freq_index = act_freq_index;
        imu_act_imagpart = act_complexpart; 
%         one_locus_set(act_freq_index,INDEX_IMAGPART,act_cellno)=...
%             act_complexpart;
%         
        imu_request_succed=true; % both received ready
%         gateway_request(IMU) = false;
        next_gateway_request =true;
    end
    
elseif(imu_request == IMU_POLLING)
    status = uint16(bitand(uint32(hex2dec('000000FF')),...
            bitshift(msg(1),-8)));
    if (status == uint16(1))
        imu_mfc_ready = true;
    else
        imu_mfc_ready = false;
    end
    imu_request_succed=true;
%     gateway_request(IMU) = false;
    next_gateway_request =true;
    
elseif(imu_request == IMU_OFFSET_POLLING)
    status = uint16(bitand(uint32(hex2dec('000000FF')),...
            bitshift(msg(1),-8)));
    if (status == uint16(1))
        imu_offset_ready = true;
    else
        imu_offset_ready = false;
    end
    imu_request_succed=true;
%     gateway_request(IMU) = false;
    next_gateway_request =true;
    
elseif(imu_request == IMU_AMP_OFF)
    
   offset_imu  = uint16(bitand(uint32(hex2dec('0000FFFF')),...
            bitshift(msg(1),-16)));
   amplitude_imu = uint16(bitand(uint32(hex2dec('0000FFFF')),msg(2)));
    if((amplitude_imu == imu_amplitude) && (offset_imu == imu_offset))
       imu_request_succed=true;
%        gateway_request(IMU) = false;
       next_gateway_request =true;
    else
        gateway_request(IMU) = true;
    end
    
elseif imu_request == imu_id
       imu_request_succed=true;
%        gateway_request(IMU) = false;
       next_gateway_request =true;
end

== stateflow chart BMS_V4/Statemachine ==
  state switch_off
    en:
    information_mode =  SHUT_DOWN_BALANCE_OFF;
    gateway_request[INFO - uint16(1)] = true;
  state Save_soc
    en:
    mram_command[SOC_CC_STORE-uint16(1)]=true;
  state start_IMU_SCC
    state scc_requierd
      en:
      led1=true;
      //CANA_send_data[SYSTEM_DEBUG - uint16(1)] = true;
    state Current_Control
      en:
      contactor_request = true;
      gateway_request[ CONTACTOR - uint16(1)] = true;
    state meas_locus
      state led_off
        en:
        led1=false;
      state led_on
        en:
        led1=true;
      start_IMU_SCC.meas_locus.led_off -> start_IMU_SCC.meas_locus.led_on [order 1] : after(single(0.5),sec)
      start_IMU_SCC.meas_locus.led_on -> start_IMU_SCC.meas_locus.led_off [order 1] : after(single(0.5),sec)
      start_IMU_SCC.meas_locus.led_off -> (junction 143) [order 2] : [imu_finish==true]
      start_IMU_SCC.meas_locus.led_on -> (junction 143) [order 2] : [imu_finish==true]
    state contactor_on
      contactor1=false;
    (default) -> scc_requierd
    start_IMU_SCC.contactor_on -> start_IMU_SCC.meas_locus.led_off : after(single(1),sec)
        | {imu_function = START_IMU_SCC;}
    scc_requierd -> start_IMU_SCC.Current_Control : //[(abs(line_currents)<IMU_LINE_CURRENT_THRESHHOLD) && ...
        | //(soc_ref_enable == true) &&...
        | //(CANA_send_data[SYSTEM_DEBUG - uint16(1)] == false)]
        | [abs(line_currents)<IMU_LINE_CURRENT_THRESHHOLD]
    start_IMU_SCC.Current_Control -> start_IMU_SCC.contactor_on : [contactor_unlocked == true]
  state Master_init
    en:
    //load mram data
    mram_command[SOC_CC_READ-uint16(1)]=true;
    mram_command[SOC_ABS_READ-uint16(1)]=true;
    mram_command[SOC_SCC_READ - uint16(1)]= true;
    mram_command[READ_LAST_SOC_INDEX_SCC - uint16(1)]= true;
  state Master_ready
    en:
    balance_flag = true;
    contactor1=true;
    soc_ref_required = false;
    soc_ref_in_progress = false;
    //CANA_send_data[SYSTEM_DEBUG - uint16(1)] = true;
    exit:
    balance_flag = false;
  state correct_current
    en:
    //activate_current_correction=true;
  state contactor
    en:
    contactor_request = true;
    gateway_request[ CONTACTOR - uint16(1)] = true;
  state Manual_imu_requierd
    en:
    user_imu_request=false;
    system_function[MANUAL_SOC_OCV_REF -uint16(1)] =false;
    led1=true;
    system_debug_request = REQUEST_SOC_REF;
    soc_ref_required = true;
    //CANA_send_data[SYSTEM_DEBUG - uint16(1)] = true;
  state Balance_Charge_Activate
    state Ready
      en:
      gateway_request[ BALANCE - uint16(1)] = true;
    state wait
    state Balancing_control
      en:
      balance_vector = BALANCE_VECTOR_INIT;
      gateway_request[ BALANCE - uint16(1)] = true;
    Ready -> wait
    wait -> (junction 182) : after(2,sec)
        | [gateway_request[ BALANCE - uint16(1)] == false]
    (junction 182) -> Ready [order 2]
    (junction 182) -> Balancing_control [order 1] : [system_function[BALANCE_CHARGE -uint16(1)] == false]
  state reset_soc_abs
    en:
    led1=false;
    cell_soc_ABS = int32(0);
    //contactor1=false;
    system_debug_request = REQUEST_SOC_REF;
    soc_ref_required = false;
    soc_ref_in_progress = false;
    //CANA_send_data[SYSTEM_DEBUG - uint16(1)] = true;
  state Current_Control
    en:
    contactor_request = true;
    gateway_request[ CONTACTOR - uint16(1)] = true;
  state meas_locus
    state led_off
      en:
      led1=false;
    state led_on
      en:
      led1=true;
    meas_locus.led_off -> meas_locus.led_on [order 1] : after(single(0.5),sec)
    meas_locus.led_on -> meas_locus.led_off [order 1] : after(single(0.5),sec)
    meas_locus.led_off -> (junction 44) [order 2] : [imu_finish==true]
    meas_locus.led_on -> (junction 44) [order 2] : [imu_finish==true]
  state contactor_on
    contactor1=false;
    soc_ref_in_progress = true;
    system_debug_request = REQUEST_SOC_REF;
    //CANA_send_data[SYSTEM_DEBUG - uint16(1)] = true;
  state wait_imu
  state ref_ocv
    state wait_1h
      en:
      led1 = true;
      %du:
      %led2 = not(led2);
    state start_ref
      en:
      soc_ref_required = false;
      soc_ocv_ref();
      system_debug_request = REQUEST_SOC_REF;
      CANA_send_data[SYSTEM_DEBUG - uint16(1)] = true;
    wait_1h -> start_ref : after(TIMER_OCV_REF,sec)
  Balancing_control -> Master_ready : [gateway_request[ BALANCE - uint16(1)] == false]
      | {led2 = false;}
  Master_ready -> Ready [order 4] : [system_function[BALANCE_CHARGE -uint16(1)] == true]
      | {led2 = true;}
  wait_imu -> meas_locus.led_off : after(single(1),sec)
      | {//activate_current_correction = true;
      | imu_function = START_IMU_MSL;}
  Save_soc -> switch_off : //after(5,sec)...
      | [mram_command[SOC_CC_STORE-uint16(1)] == false]
  (junction 72) -> wait_1h [order 1] : [REF_IMU_OR_OCV > uint16(0)]
  (junction 44) -> reset_soc_abs
  start_ref -> reset_soc_abs : [after(single(5),sec) &&...
      |  CANA_send_data[SYSTEM_DEBUG - uint16(1)] == false]
  (junction 143) -> Master_ready : {led1=false;}
  Master_ready -> Save_soc [order 2] : [system_function[HARDWARE_RESET -uint16(1)] == true]
  (default) -> Master_init
  Master_ready -> start_IMU_SCC [order 3] : [user_imu_request == START_IMU_SCC]
      | {user_imu_request = uint16(0)}
      | //reset user_imu_request
  contactor -> correct_current : [contactor_unlocked == true]
  correct_current -> Master_ready : [activate_current_correction==false]
  Master_init -> contactor : after(TIMER_MASTER_INIT,sec)
  reset_soc_abs -> Master_ready : [CANA_send_data[SYSTEM_DEBUG - uint16(1)] == false]
  Master_ready -> Manual_imu_requierd [order 1] : [(cell_soc_ABS > MEAS_LOCUS_SOC_LIMIT) || (user_imu_request == START_IMU_MSL) ||...
      | system_function[MANUAL_SOC_OCV_REF -uint16(1)] == true]
      | {user_imu_request = uint16(0)}
      | //reset user_imu_request
  Manual_imu_requierd -> Current_Control : //[(abs(line_currents)<IMU_LINE_CURRENT_THRESHHOLD) && ...
      | //(soc_ref_enable == true) &&...
      | //(CANA_send_data[SYSTEM_DEBUG - uint16(1)] == false)]
      | [abs(line_currents)<IMU_LINE_CURRENT_THRESHHOLD]
  Current_Control -> contactor_on : [contactor_unlocked == true]
  contactor_on -> (junction 72) : [CANA_send_data[SYSTEM_DEBUG - uint16(1)] == false]
  (junction 72) -> wait_imu [order 2] : [REF_IMU_OR_OCV == uint16(0)]
  data: TIMER_MASTER_INIT parameter; cell_soc_ABS data_store_memory; MEAS_LOCUS_SOC_LIMIT parameter; led1 output =false; START_IMU_MSL parameter; imu_function data_store_memory; imu_finish data_store_memory; CONTACTOR parameter; gateway_request data_store_memory; contactor_unlocked data_store_memory; contactor_request data_store_memory; user_imu_request data_store_memory; IMU_LINE_CURRENT_THRESHHOLD parameter; line_currents data_store_memory; activate_current_correction data_store_memory; SOC_CC_READ parameter; mram_command data_store_memory; REF_IMU_OR_OCV parameter; TIMER_OCV_REF parameter; soc_ref_enable data_store_memory; soc_ref_required data_store_memory; soc_ref_in_progress data_store_memory; cell_soc_CC data_store_memory; system_debug_request data_store_memory; REQUEST_SOC_REF parameter; SYSTEM_DEBUG parameter; CANA_send_data data_store_memory; system_function data_store_memory; MANUAL_SOC_OCV_REF parameter; HARDWARE_RESET parameter; information_mode data_store_memory; SHUT_DOWN_BALANCE_OFF parameter; INFO parameter; SOC_CC_STORE parameter; START_IMU_SCC parameter; max_cell_voltage data_store_memory; BALANCE_CHARGE_V_CELL_MAX parameter; BALANCE_CHARGE parameter; led2 output =false; contactor1 output; balance_vector data_store_memory; cell_voltages data_store_memory; BALANCE parameter; BALANCE_VECTOR_INIT parameter size=[NUM_OF_CELLS,NUM_OF_LINES]; NUM_OF_CELLS parameter; SOC_ABS_READ parameter; SOC_SCC_READ parameter; READ_LAST_SOC_INDEX_SCC parameter; balance_flag data_store_memory
  events: trigger_Statemachine input FUNCTION_CALL_EVENT
  function soc_ocv_ref:
    | function soc_ocv_ref()
    | 
    | global cell_soc_CC;
    | 
    | cell_soc_CC(2,1) = int32(55*1e6);
    | 
    | end
